simulink model "linmodel_eq2_lqr"  (R2019a)
settings: Solver=VariableStepAuto  StartTime=0.0  StopTime=10.0  RelTol=1e-3
values from neighbouring files (symbols this model uses):
  A_eq2 = [0 0 1 0 ... (first row only)    [lin_discr_model.m]
  B = [0 0 ... (first row only)    [lin_discr_model.m]
  C = [1 0 0 0 ... (first row only)    [lin_discr_model.m]
undefined symbols (not defined in the file or in its folder): Continuous, K2, matrcomp, par, Time
libraries: ctrlSharedLib x1
settings Model: Creator=jessi  LastModifiedBy=jessi

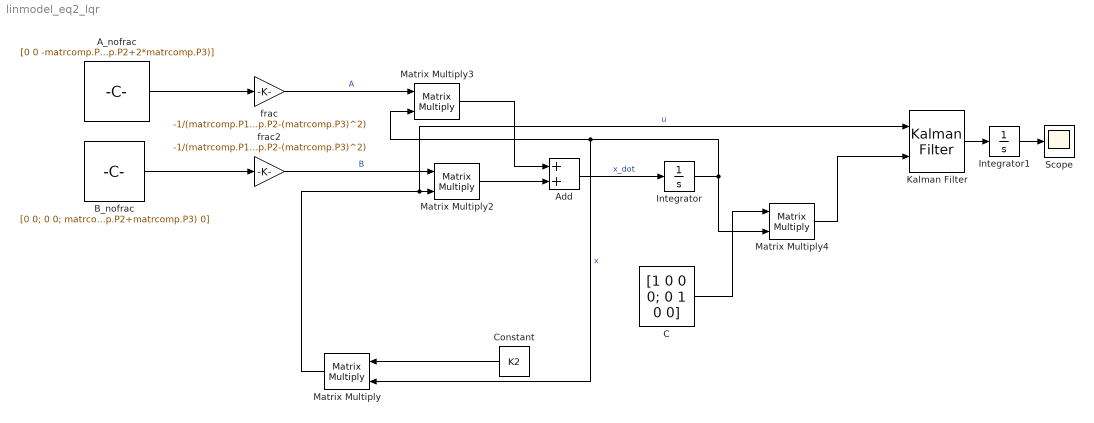
== system linmodel_eq2_lqr ==
  A_nofrac : Constant  Value=[0 0 -matrcomp.P1*matrcomp.P2+(matrcomp.P3)^2 0; 0 0 0 -matrcomp.P1*matrcomp.P2+(matrcomp.P3)^2; -matrcomp.g1*matrcomp.P2+matrcomp.g2*matrcomp.P3 matrcomp.g2*matrcomp.P3 par.b1*matrcomp.P2 -par.b2*(matrcomp.P2+matrcomp.P3); matrcomp.g1*(matrcomp.P2+matrcomp.P3)-matrcomp.g2*(matrcomp.P1+matrcomp.P3) -matrcomp.g2*(matrcomp.P1+matrcomp.P3) -par.b1*(matrcomp.P2+matrcomp.P3) par.b2*(matrcomp.P1+matrcomp.P2+2*matrcomp.P3)]
  Add : Sum
  B_nofrac : Constant  Value=[0 0; 0 0; matrcomp.P2*par.km 0; -par.km*(matrcomp.P2+matrcomp.P3) 0]
  C : Constant  Value=|
      | [1 0 0 0;
      | 0 1 0 0]
  Constant : Constant  Value=K2
  Integrator : Integrator
  Integrator1 : Integrator
  Kalman Filter : ctrlSharedLib/Kalman Filter  TimeDomain=Continuous-Time  UseCurrentEstimator=on  ModelSource=Individual A, B, C, D matrices  ModelSourceVariable=ss(0.95,1,1,0,1)  A=A_eq2  B=B  C=C  D=0  NumberOfStates=1  NumberOfInputs=1  NumberOfOutputs=1  InitialEstimateSource=Dialog  X0=[pi;0;0;0]  P0=10  UseK=off  UseGH=off  NumberOfProcessNoiseInputs=1  G=1  TimeInvariantG=on  H=0  TimeInvariantH=on  Q=0.05  TimeInvariantQ=on  R=1  TimeInvariantR=on  N=0  TimeInvariantN=on  AddInputPort=on  AddEnablePort=off  OutputEstimatedY=off  OutputP=off  Ts=-1
      settings: SourceProductBaseCode=CT
  Matrix Multiply{,2..4} (4 alike) : Product  Multiplication=Matrix(*)
  Scope : Scope
  frac : Gain  Gain=-1/(matrcomp.P1*matrcomp.P2-(matrcomp.P3)^2)
  frac2 : Gain  Gain=-1/(matrcomp.P1*matrcomp.P2-(matrcomp.P3)^2)
  wires:
  frac2/1 -> Matrix Multiply2/1  "B"
  Matrix Multiply2/1 -> Add/2
  frac/1 -> Matrix Multiply3/1  "A"
  Add/1 -> Integrator/1  "x_dot"
  Integrator/1 -> Matrix Multiply4/2, Matrix Multiply3/2, Matrix Multiply/2  "x"
  Matrix Multiply3/1 -> Add/1
  A_nofrac/1 -> frac/1
  B_nofrac/1 -> frac2/1
  C/1 -> Matrix Multiply4/1
  Matrix Multiply/1 -> Kalman Filter/1, Matrix Multiply2/2  "u"
  Constant/1 -> Matrix Multiply/1
  Integrator1/1 -> Scope/1
  Matrix Multiply4/1 -> Kalman Filter/2
  Kalman Filter/1 -> Integrator1/1
